simulink model "TestDatacenter"  (R2025a)
settings: Solver=daessc  StartTime=0.0  StopTime=3600*24  FixedStep=3600  MaxStep=3600  RelTol=1e-3  AbsTol=1e-3
libraries: fl_lib x33, Datacenter_lib x6, ee_lib x3, nesl_utility x2, ThreePhaseLoad_lib x1
settings Model: Creator=vikrants  LastModifiedBy=vikrants
settings SolverCC: AutoScaleAbsTol=off  AlgebraicLoopSolver=TrustRegion  MaxZcPerStep=1.0
settings DebuggingCC: UnconnectedInputMsg=warning  UnconnectedOutputMsg=warning  UnconnectedLineMsg=warning  SymbolicDimsDataTypeCodeGenerationDiagnostic=none
settings ModelReferenceCC: EnableRefExpFcnMdlSchedulingChecks=on
settings SFSimCC: CustomCodeUndefinedFunction=UseInterfaceOnly
settings RTWCC: GPUComputeCapability=3.5  DLArmComputeVersion=19.05
settings SimscapeCC: SimscapeLogLimitData=off  SimscapeLogDataHistory=10000.0  SimscapeCompileComponentReuse=on

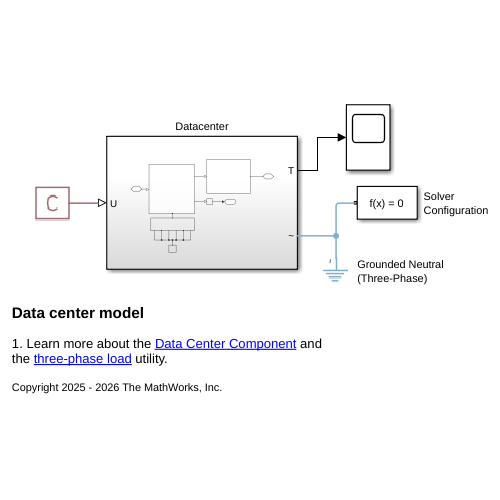
[thumbnail: Simulink's stored preview of the top-level diagram]
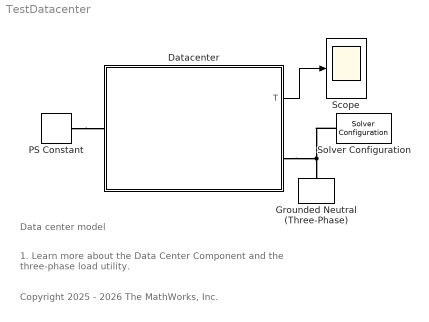
== system TestDatacenter ==
  note: Copyright 2025 - 2026 The MathWorks, Inc.
  note: Data center model
  note: 1. Learn more about the Data Center Component and
      | the three-phase load utility.
  Datacenter : Subsystem
  Grounded Neutral (Three-Phase) : ee_lib/Connectors & References/Grounded Neutral (Three-Phase)
  PS Constant : fl_lib/Physical Signals/Sources/PS Constant  constant=[0.5 0.6 0.4 0.55 0.45 0.25]
  Scope : Scope
      settings: ActiveDisplayYMinimum=299.62151119325034  ActiveDisplayYMaximum=300.04205431186108
  Solver Configuration : nesl_utility/Solver Configuration  PhysicalDomain=network_engine_domain  SubClassName=solver  LeftPortType=input  RightPortType=generic  Tones=[]  Harmonics=[]  SimulateNoise=off  Profile=off  UseLocalSampling=off  EnableSwitchedLinearOptims=on  FrequencyDomain=off  UseCCode=off  RelTol=0.001  AbsTol=1e-06  MinStep=1e-09  ToWorkspace=off  RevertToSquareIcSolve=off  NumHomotopyIterations=100  PhasorMode=off  PhasorModeNumHarmonics=1  ConsistencySolver=NEWTON_XTOL_AFTER_FTOL  IndexReductionMethod=DerivativeReplacement  DoDC=off  ResidualTolerance=1e-09  ConsistencyTolSource=GLOBAL  ConsistencyAbsTol=0.001  ConsistencyRelTol=0.001  ConsistencyTolFactor=0.001  UseLocalSolver=off  LocalSolverChoice=NE_BACKWARD_EULER_ADVANCER  ResolveIndetEquations=on  FunctionEvalNumThread=1  LocalSolverSampleTime=0.001  DoFixedCost=off  MaxNonlinIter=3  MaxModeIter=2  ComputeImpulses=off  ImpulseIterations=2  LinearAlgebra=auto  LinearAlgebraNumThread=0  EquationFormulation=NE_TIME_EF  DelaysMemoryBudget=1024  AutomaticFiltering=on  FilteringTimeConstant=0.001  PartitionStorageMethod=AS_NEEDED  PartitionMemoryBudget=1024  PartitionMethod=ROBUST  MultibodyUseLocalSolver=off  MultibodyLocalSolverChoice=ODE1  MultibodyLocalSolverSampleTime=0.001
  wires:
  Datacenter/1(T) -> Scope/1
  connections:
  Datacenter/RConn1 -- Grounded Neutral (Three-Phase)/LConn1 -- Solver Configuration/RConn1
  PS Constant/RConn1 -- Datacenter/LConn1

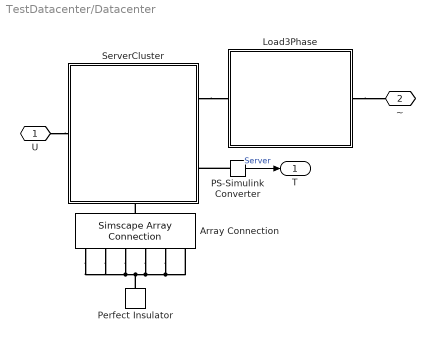
== system TestDatacenter/Datacenter ==
  Array Connection : SimscapeArrayConnection  Domain=foundation.thermal.thermal  ConcatenateDimension=1  NumScalarElements=6
  Load3Phase : Subsystem
  PS-Simulink Converter : nesl_utility/PS-Simulink Converter  PhysicalDomain=network_engine_domain  SubClassName=ps_output  LeftPortType=input  RightPortType=output  PseudoPeriodic=off  Frequencies=[]  VectorFormat=inherit  Unit=inherit  AffineConversion=off
  Perfect Insulator : fl_lib/Thermal/Thermal Elements/Perfect Insulator  T_specify=off  T_priority=None  T=293.15 K  T_nominal_specify=off  T_nominal_value=1  T_nominal_unit=K
  ServerCluster : Subsystem
      settings: PortSchema="{\"entries\":[{\"content\":{\"sides\":[{\"content\":{\"connectorIds\":[\"LConn1\"]},\"type\":\"ConnectorPlacement.EquallySpacedRectSide\",\"uuid\":\"e6fad092-4fff-4871-b130-bfab87c2e174\"},{\"content\":{\"connectorIds\":[\"RConn1\",\"RConn2\"],\"side\":\"RIGHT\"},\"type\":\"ConnectorPlacement.EquallySpacedRectSide\",\"uuid\":\"8860b590-9823-4650-a297-c38cc87365c3\"},{\"content\":{\"side\":\"TOP\"},\"type\":\"ConnectorPlacement.EquallySpacedRectSide\",\"uuid\":\"a53cafe0-870d-4f25-a9a4-7a34c2d7c09f\"},{\"content\":{\"connectorIds\":[\"RConn3\"],\"side\":\"BOTTOM\"},\"type\":\"ConnectorPlacement.EquallySpacedRectSide\",\"uuid\":\"f820ad35-c8ec-43d2-9d29-396c0291562e\"}]},\"type\":\"ConnectorPlacement.EquallySpacedConnector\",\"uuid\":\"402250ae-721f-4c4a-9a90-f63e45e66938\"}],\"packageUris\":[\"http://schema.mathworks.com/mf0/Connector/R2020b\"],\"version\":\"1.0\"}"
  U : PMIOPort  Side=Left
  ~ : PMIOPort  Port=2  Side=Right
  T : Outport
  wires:
  PS-Simulink Converter/1 -> T/1  "Server"
  connections:
  Load3Phase/RConn1 -- ~/RConn1
  PS-Simulink Converter/LConn1 -- ServerCluster/RConn2
  U/RConn1 -- ServerCluster/LConn1
  ServerCluster/RConn1 -- Load3Phase/LConn1
  Perfect Insulator/LConn1 -- Array Connection/LConn2 -- Array Connection/LConn1 -- Array Connection/LConn3 -- Array Connection/LConn5 -- Array Connection/LConn6 -- Array Connection/LConn4
  Array Connection/RConn1 -- ServerCluster/RConn3

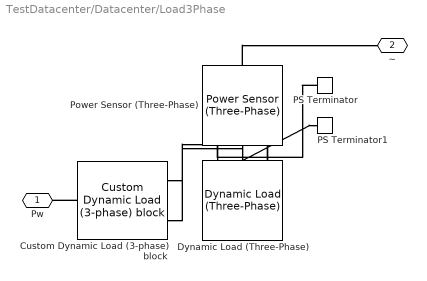
== system TestDatacenter/Datacenter/Load3Phase ==
  Custom Dynamic Load (3-phase) block : ThreePhaseLoad_lib/Custom Dynamic Load (3-phase) block  Pf=.98  THD=0  N=6
      settings: InternalSimscapePortConfiguration="{\"Bottom\":[],\"Left\":[{\"id\":\"Pw\",\"label\":\"Pvec\",\"type\":\"input\"}],\"Right\":[{\"id\":\"P\",\"label\":\"P\",\"type\":\"output\"},{\"id\":\"Q\",\"label\":\"Q\",\"type\":\"output\"}],\"Top\":[]}"
  Dynamic Load (Three-Phase) : ee_lib/Passive/Dynamic Load (Three-Phase)  port_option=ee.enum.threePhasePort.composite  FRated=60 Hz  Vline_rms_min=100 V  tau=0.01 s  Vline_rms_ini=200 V  Vang_ini=0 deg  gmin=0 S
      settings: InternalSimscapePortConfiguration="{\"Bottom\":[],\"Left\":[{\"id\":\"N\",\"label\":\"~\",\"type\":\"foundation.electrical.three_phase\"}],\"Right\":[],\"Top\":[{\"id\":\"P\",\"label\":\"P\",\"type\":\"input\"},{\"id\":\"Q\",\"label\":\"Q\",\"type\":\"input\"}]}"
  PS Terminator : fl_lib/Physical Signals/Sinks/PS Terminator
  PS Terminator1 : fl_lib/Physical Signals/Sinks/PS Terminator
  Power Sensor (Three-Phase) : ee_lib/Sensors & Transducers/Power Sensor (Three-Phase)  load_type=ee.enum.passive.type_balanced.balanced  f0=60 Hz  config=ee.enum.with_neutral.no  rho=1
      settings: InternalSimscapePortConfiguration="{\"Bottom\":[],\"Left\":[{\"id\":\"N1\",\"label\":\"~1\",\"type\":\"foundation.electrical.three_phase\"}],\"Right\":[{\"id\":\"N2\",\"label\":\"~2\",\"type\":\"foundation.electrical.three_phase\"}],\"Top\":[{\"id\":\"Pm\",\"label\":\"P\",\"type\":\"output\"},{\"id\":\"Qm\",\"label\":\"Q\",\"type\":\"output\"}]}"
  Pw : PMIOPort  Side=Left
  ~ : PMIOPort  Port=2  Side=Right
  connections:
  Custom Dynamic Load (3-phase) block/RConn1 -- Dynamic Load (Three-Phase)/LConn2
  Custom Dynamic Load (3-phase) block/RConn2 -- Dynamic Load (Three-Phase)/LConn3
  Power Sensor (Three-Phase)/LConn1 -- Dynamic Load (Three-Phase)/LConn1
  Power Sensor (Three-Phase)/RConn1 -- ~/RConn1
  Custom Dynamic Load (3-phase) block/LConn1 -- Pw/RConn1
  PS Terminator/LConn1 -- Power Sensor (Three-Phase)/LConn3
  Power Sensor (Three-Phase)/LConn2 -- PS Terminator1/LConn1

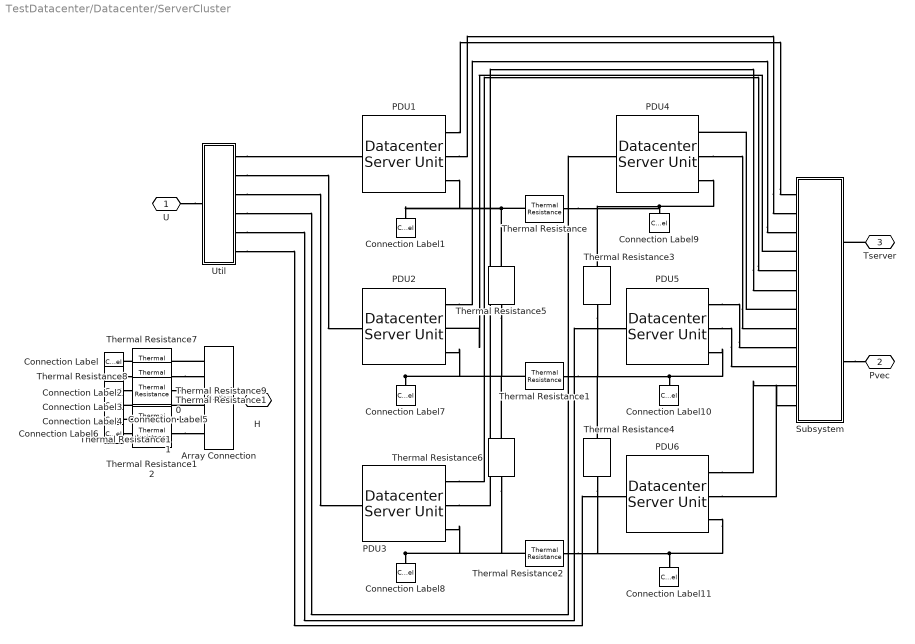
== system TestDatacenter/Datacenter/ServerCluster ==
  Array Connection : SimscapeArrayConnection  Domain=foundation.thermal.thermal  ConcatenateDimension=1  NumScalarElements=6
  Connection Label : ConnectionLabel  Label=dc1
  Connection Label1 : ConnectionLabel  Label=dc1
  Connection Label10 : ConnectionLabel  Label=dc5
  Connection Label11 : ConnectionLabel  Label=dc6
  Connection Label2 : ConnectionLabel  Label=dc2
  Connection Label3 : ConnectionLabel  Label=dc3
  Connection Label4 : ConnectionLabel  Label=dc4
  Connection Label5 : ConnectionLabel  Label=dc5
  Connection Label6 : ConnectionLabel  Label=dc6
  Connection Label7 : ConnectionLabel  Label=dc2
  Connection Label8 : ConnectionLabel  Label=dc3
  Connection Label9 : ConnectionLabel  Label=dc4
  PDU{1..6} (6 alike) : Datacenter_lib/Datacenter Server Unit  peakPowCPU=40 W  numOfCPU=2  peakPowMemory=9 W  numOfMemory=4  peakPowDisk=12 W  numOfDisk=1  peakPowPCIslot=25 W  numOfPCIslot=2  peakPowMotherboard=25 W  numOfMotherboard=1  peakPowFan=10 W  numOfFan=1  powerSupplyEff=85  numCPUperServer=20  ratioActualToNameplate=0.6  serverMass=1 kg  serverSpHeat=2500 J/(K*kg)  idlePower=25 W  physQ=datacenterPhysics.linear  calibParam=1  T_specify=off  T_priority=High  T=300 K  T_nominal_specify=off  T_nominal_value=1  T_nominal_unit=K  Q_specify=off  Q_priority=None  Q=0 W  Q_nominal_specify=off  Q_nominal_value=1  Q_nominal_unit=W
      settings: InternalSimscapePortConfiguration="{\"Bottom\":[{\"id\":\"H\",\"label\":\"H\",\"type\":\"foundation.thermal.thermal\"}],\"Left\":[{\"id\":\"U\",\"label\":\"U\",\"type\":\"input\"}],\"Right\":[{\"id\":\"To\",\"label\":\"T\",\"type\":\"output\"},{\"id\":\"P\",\"label\":\"P\",\"type\":\"output\"}],\"Top\":[]}"
  Subsystem : Subsystem
  Thermal Resistance{,1..6} (7 alike) : fl_lib/Thermal/Thermal Elements/Thermal Resistance  resistance=1000 K/W  T_specify=off  T_priority=None  T=0 K  T_nominal_specify=off  T_nominal_value=1  T_nominal_unit=K  Q_specify=off  Q_priority=None  Q=0 W  Q_nominal_specify=off  Q_nominal_value=1  Q_nominal_unit=W
  Thermal Resistance{7..12} (6 alike) : fl_lib/Thermal/Thermal Elements/Thermal Resistance  resistance=0.01 K/W  T_specify=off  T_priority=None  T=0 K  T_nominal_specify=off  T_nominal_value=1  T_nominal_unit=K  Q_specify=off  Q_priority=None  Q=0 W  Q_nominal_specify=off  Q_nominal_value=1  Q_nominal_unit=W
  Util : Subsystem
  U : PMIOPort  Side=Left
  Pvec : PMIOPort  Port=2  Side=Right
  Tserver : PMIOPort  Port=3  Side=Right
  H : PMIOPort  Port=4  Side=Right
  connections:
  Thermal Resistance5/LConn1 -- PDU1/RConn3 -- Connection Label1/LConn1 -- Thermal Resistance/LConn1
  Thermal Resistance8/LConn1 -- Array Connection/LConn2
  Thermal Resistance5/RConn1 -- Thermal Resistance6/LConn1 -- Thermal Resistance1/LConn1 -- PDU2/RConn3 -- Connection Label7/LConn1
  Thermal Resistance2/LConn1 -- Thermal Resistance6/RConn1 -- PDU3/RConn3 -- Connection Label8/LConn1
  Thermal Resistance/RConn1 -- Thermal Resistance3/LConn1 -- PDU4/RConn3 -- Connection Label9/LConn1
  Thermal Resistance1/RConn1 -- Thermal Resistance3/RConn1 -- Thermal Resistance4/LConn1 -- PDU5/RConn3 -- Connection Label10/LConn1
  Thermal Resistance4/RConn1 -- Thermal Resistance2/RConn1 -- Connection Label11/LConn1 -- PDU6/RConn3
  Thermal Resistance7/RConn1 -- Connection Label/LConn1
  Connection Label3/LConn1 -- Thermal Resistance9/RConn1
  Array Connection/LConn4 -- Thermal Resistance10/LConn1
  Array Connection/LConn5 -- Thermal Resistance11/LConn1
  Connection Label6/LConn1 -- Thermal Resistance12/RConn1
  Array Connection/RConn1 -- H/RConn1
  Array Connection/LConn1 -- Thermal Resistance7/LConn1
  Connection Label2/LConn1 -- Thermal Resistance8/RConn1
  Thermal Resistance9/LConn1 -- Array Connection/LConn3
  Thermal Resistance10/RConn1 -- Connection Label4/LConn1
  Thermal Resistance11/RConn1 -- Connection Label5/LConn1
  Thermal Resistance12/LConn1 -- Array Connection/LConn6
  Util/RConn1 -- PDU1/LConn1
  Util/RConn4 -- PDU4/LConn1
  U/RConn1 -- Util/LConn1
  Util/RConn2 -- PDU2/LConn1
  Util/RConn5 -- PDU5/LConn1
  Util/RConn6 -- PDU6/LConn1
  Util/RConn3 -- PDU3/LConn1
  Tserver/RConn1 -- Subsystem/RConn1
  Subsystem/RConn2 -- Pvec/RConn1
  PDU1/RConn1 -- Subsystem/LConn1
  PDU1/RConn2 -- Subsystem/LConn2
  PDU2/RConn1 -- Subsystem/LConn3
  Subsystem/LConn4 -- PDU2/RConn2
  PDU3/RConn1 -- Subsystem/LConn5
  PDU3/RConn2 -- Subsystem/LConn6
  Subsystem/LConn7 -- PDU4/RConn1
  PDU4/RConn2 -- Subsystem/LConn8
  PDU5/RConn1 -- Subsystem/LConn9
  PDU5/RConn2 -- Subsystem/LConn10
  PDU6/RConn1 -- Subsystem/LConn11
  PDU6/RConn2 -- Subsystem/LConn12

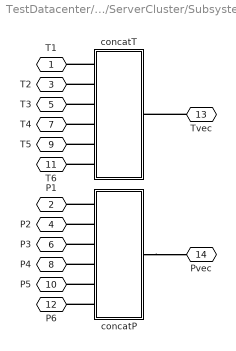
== system TestDatacenter/Datacenter/ServerCluster/Subsystem ==
  concatP : Subsystem
  concatT : Subsystem
  T1 : PMIOPort  Side=Left
  P1 : PMIOPort  Port=2  Side=Left
  T2 : PMIOPort  Port=3  Side=Left
  P2 : PMIOPort  Port=4  Side=Left
  T3 : PMIOPort  Port=5  Side=Left
  P3 : PMIOPort  Port=6  Side=Left
  T4 : PMIOPort  Port=7  Side=Left
  P4 : PMIOPort  Port=8  Side=Left
  T5 : PMIOPort  Port=9  Side=Left
  P5 : PMIOPort  Port=10  Side=Left
  T6 : PMIOPort  Port=11  Side=Left
  P6 : PMIOPort  Port=12  Side=Left
  Tvec : PMIOPort  Port=13  Side=Right
  Pvec : PMIOPort  Port=14  Side=Right
  connections:
  concatT/LConn3 -- T3/RConn1
  concatP/RConn1 -- Pvec/RConn1
  concatP/LConn2 -- P2/RConn1
  Tvec/RConn1 -- concatT/RConn1
  concatP/LConn4 -- P4/RConn1
  concatP/LConn1 -- P1/RConn1
  concatP/LConn5 -- P5/RConn1
  concatT/LConn1 -- T1/RConn1
  concatT/LConn2 -- T2/RConn1
  concatT/LConn6 -- T6/RConn1
  concatP/LConn3 -- P3/RConn1
  concatP/LConn6 -- P6/RConn1
  concatT/LConn5 -- T5/RConn1
  concatT/LConn4 -- T4/RConn1

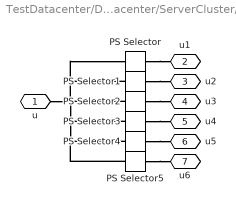
== system TestDatacenter/Datacenter/ServerCluster/Util ==
  PS Selector : fl_lib/Physical Signals/Nonlinear Operators/PS Selector  ix=1
      settings: InternalSimscapePortConfiguration="{\"Bottom\":[],\"Left\":[{\"id\":\"I\",\"label\":\"\",\"type\":\"input\"}],\"Right\":[{\"id\":\"O\",\"label\":\"\",\"type\":\"output\"}],\"Top\":[]}"
  PS Selector1 : fl_lib/Physical Signals/Nonlinear Operators/PS Selector  ix=2
      settings: InternalSimscapePortConfiguration="{\"Bottom\":[],\"Left\":[{\"id\":\"I\",\"label\":\"\",\"type\":\"input\"}],\"Right\":[{\"id\":\"O\",\"label\":\"\",\"type\":\"output\"}],\"Top\":[]}"
  PS Selector2 : fl_lib/Physical Signals/Nonlinear Operators/PS Selector  ix=3
      settings: InternalSimscapePortConfiguration="{\"Bottom\":[],\"Left\":[{\"id\":\"I\",\"label\":\"\",\"type\":\"input\"}],\"Right\":[{\"id\":\"O\",\"label\":\"\",\"type\":\"output\"}],\"Top\":[]}"
  PS Selector3 : fl_lib/Physical Signals/Nonlinear Operators/PS Selector  ix=4
      settings: InternalSimscapePortConfiguration="{\"Bottom\":[],\"Left\":[{\"id\":\"I\",\"label\":\"\",\"type\":\"input\"}],\"Right\":[{\"id\":\"O\",\"label\":\"\",\"type\":\"output\"}],\"Top\":[]}"
  PS Selector4 : fl_lib/Physical Signals/Nonlinear Operators/PS Selector  ix=5
      settings: InternalSimscapePortConfiguration="{\"Bottom\":[],\"Left\":[{\"id\":\"I\",\"label\":\"\",\"type\":\"input\"}],\"Right\":[{\"id\":\"O\",\"label\":\"\",\"type\":\"output\"}],\"Top\":[]}"
  PS Selector5 : fl_lib/Physical Signals/Nonlinear Operators/PS Selector  ix=6
      settings: InternalSimscapePortConfiguration="{\"Bottom\":[],\"Left\":[{\"id\":\"I\",\"label\":\"\",\"type\":\"input\"}],\"Right\":[{\"id\":\"O\",\"label\":\"\",\"type\":\"output\"}],\"Top\":[]}"
  u : PMIOPort  Side=Left
  u1 : PMIOPort  Port=2  Side=Right
  u2 : PMIOPort  Port=3  Side=Right
  u3 : PMIOPort  Port=4  Side=Right
  u4 : PMIOPort  Port=5  Side=Right
  u5 : PMIOPort  Port=6  Side=Right
  u6 : PMIOPort  Port=7  Side=Right
  connections:
  PS Selector1/RConn1 -- u2/RConn1
  PS Selector2/RConn1 -- u3/RConn1
  PS Selector5/RConn1 -- u6/RConn1
  PS Selector3/RConn1 -- u4/RConn1
  PS Selector/RConn1 -- u1/RConn1
  PS Selector4/RConn1 -- u5/RConn1
  PS Selector1/LConn1 -- PS Selector5/LConn1 -- PS Selector4/LConn1 -- PS Selector3/LConn1 -- u/RConn1 -- PS Selector2/LConn1 -- PS Selector/LConn1

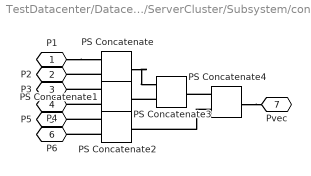
== system TestDatacenter/Datacenter/ServerCluster/Subsystem/concatP ==
  PS Concatenate{,1..4} (5 alike) : fl_lib/Physical Signals/Functions/PS Concatenate  catColumns=true
      settings: InternalSimscapePortConfiguration="{\"Bottom\":[],\"Left\":[{\"id\":\"I1\",\"label\":\"\",\"type\":\"input\"},{\"id\":\"I2\",\"label\":\"\",\"type\":\"input\"}],\"Right\":[{\"id\":\"O\",\"label\":\"\",\"type\":\"output\"}],\"Top\":[]}"
  P1 : PMIOPort  Side=Left
  P2 : PMIOPort  Port=2  Side=Left
  P3 : PMIOPort  Port=3  Side=Left
  P4 : PMIOPort  Port=4  Side=Left
  P5 : PMIOPort  Port=5  Side=Left
  P6 : PMIOPort  Port=6  Side=Left
  Pvec : PMIOPort  Port=7  Side=Right
  connections:
  P1/RConn1 -- PS Concatenate/LConn1
  PS Concatenate/LConn2 -- P2/RConn1
  PS Concatenate1/LConn1 -- P3/RConn1
  PS Concatenate1/LConn2 -- P4/RConn1
  PS Concatenate2/LConn1 -- P5/RConn1
  PS Concatenate2/LConn2 -- P6/RConn1
  PS Concatenate4/RConn1 -- Pvec/RConn1
  PS Concatenate/RConn1 -- PS Concatenate3/LConn1
  PS Concatenate3/LConn2 -- PS Concatenate1/RConn1
  PS Concatenate4/LConn1 -- PS Concatenate3/RConn1
  PS Concatenate4/LConn2 -- PS Concatenate2/RConn1

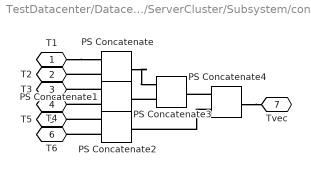
== system TestDatacenter/Datacenter/ServerCluster/Subsystem/concatT ==
  PS Concatenate{,1..4} (5 alike) : fl_lib/Physical Signals/Functions/PS Concatenate  catColumns=true
      settings: InternalSimscapePortConfiguration="{\"Bottom\":[],\"Left\":[{\"id\":\"I1\",\"label\":\"\",\"type\":\"input\"},{\"id\":\"I2\",\"label\":\"\",\"type\":\"input\"}],\"Right\":[{\"id\":\"O\",\"label\":\"\",\"type\":\"output\"}],\"Top\":[]}"
  T1 : PMIOPort  Side=Left
  T2 : PMIOPort  Port=2  Side=Left
  T3 : PMIOPort  Port=3  Side=Left
  T4 : PMIOPort  Port=4  Side=Left
  T5 : PMIOPort  Port=5  Side=Left
  T6 : PMIOPort  Port=6  Side=Left
  Tvec : PMIOPort  Port=7  Side=Right
  connections:
  T1/RConn1 -- PS Concatenate/LConn1
  PS Concatenate/LConn2 -- T2/RConn1
  PS Concatenate1/LConn1 -- T3/RConn1
  PS Concatenate1/LConn2 -- T4/RConn1
  PS Concatenate2/LConn1 -- T5/RConn1
  PS Concatenate2/LConn2 -- T6/RConn1
  PS Concatenate4/RConn1 -- Tvec/RConn1
  PS Concatenate/RConn1 -- PS Concatenate3/LConn1
  PS Concatenate3/LConn2 -- PS Concatenate1/RConn1
  PS Concatenate4/LConn1 -- PS Concatenate3/RConn1
  PS Concatenate4/LConn2 -- PS Concatenate2/RConn1
